simulink model "gsm_sms_sim900_demo"  (Simulink 7.3)
settings: Solver=FixedStepDiscrete  SolverMode=SingleTasking  StartTime=0.0  StopTime=10.0  RelTol=1e-3
PreLoadFcn:
  | waijung.modelPreload; % Required for working with Waijung Blockset. Do not remove.
undefined symbols (not defined in the file): HSEOSC, Link, LQFP176, ST, STM32F417IG
libraries: waijung_atcmd_gsmgprs_lib x2, simulink x1, stm32f4_io_lib x1, stm32f4_adc_lib x1, waijung_string_manipulate x1, stm32f4_device_config_lib x1
CloseFcn:
  | waijung.modelClose; % Required for working with Waijung Blockset. Do not remove.
settings Model: Creator=Krisada  LastModifiedBy=Krisada
settings OptimizationCC: OptimizeModelRefInitCode=on  LifeSpan=1
settings HardwareCC: ProdEndianess=LittleEndian  ProdHWDeviceType=ARM Compatible->Cortex - M4  TargetEndianess=LittleEndian  TargetHWDeviceType=ARM Compatible->Cortex - M4
settings RTWCC: SystemTargetFile=stm32f4.tlc  GenerateMakefile=off  TemplateMakefile=ert_default_tmf  Description=STM32F4 Target  ProcessScript=stm32f4_make_rtw_hook
settings CodeAppCC: IgnoreCustomStorageClasses=off
settings STFCustomTargetCC: ModelReferenceCompliant=off  CombineOutputUpdateFcns=on  ERTCustomFileBanners=on  SupportContinuousTime=off  SupportNonInlinedSFcns=off  SystemTargetFile=stm32f4.tlc
settings ERTTargetCC: MultiwordLength=2048  ModelReferenceCompliant=off  ParMdlRefBuildCompliant=off  CompOptLevelCompliant=off  ERTFirstTimeCompliant=off  ModelStepFunctionPrototypeControlCompliant=off  CPPClassGenCompliant=off  ExtModeMexFile=noextcomm  InlinedParameterPlacement=NonHierarchical  ERTSrcFileBannerTemplate=stm32f4_code_template.cgt  ERTHdrFileBannerTemplate=stm32f4_code_template.cgt  ERTDataSrcFileTemplate=stm32f4_code_template.cgt  ERTDataHdrFileTemplate=stm32f4_code_template.cgt  ERTCustomFileTemplate=stm32f4_file_process.tlc

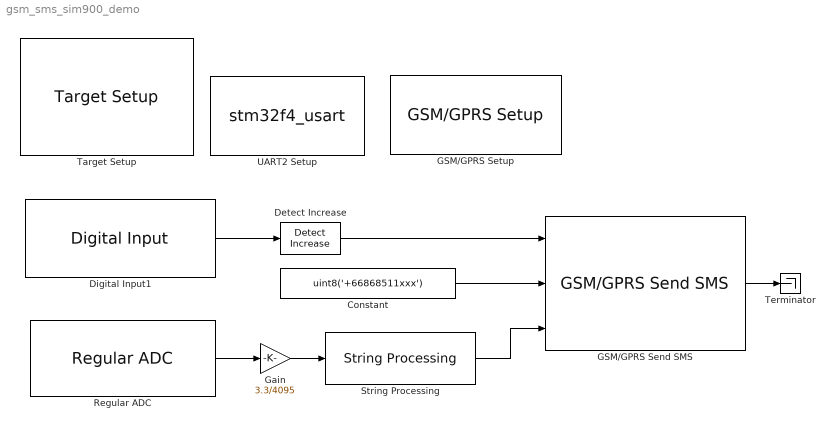
== system gsm_sms_sim900_demo ==
  Constant : Constant  Value=uint8('+66868511xxx')  OutDataType=fixdt(1, 16)  OutScaling=2^0
  Detect Increase : simulink/Logic and Bit Operations/Detect Increase  SystemSampleTime=-1  vinit=0.0
  Digital Input1 : stm32f4_io_lib/Digital Input  port=B  speed=100  porttype=None  porttypestr=NOPULL  use_pin0=off  use_pin1=off  use_pin2=on  use_pin3=off  use_pin4=off  use_pin5=off  use_pin6=off  use_pin7=off  use_pin8=off  use_pin9=off  use_pin10=off  use_pin11=off  use_pin12=off  use_pin13=off  use_pin14=off  use_pin15=off  pinstr=GPIO_Pin_2  usedpinarray="[0  0  1  0  0  0  0  0  0  0  0  0  0  0  0  0]"  bitbandingstr="#define DigitalInput1_B2 Peripheral_BB(GPIOB->IDR, 2)  /* Output pin */"  sampletime=0.01  sampletimestr=0.01  blockid=DigitalInput1  enablecustomportlabel=off  glabalinit=off  cinputportlabel=In1, In2  coutputportlabel=Out1, Out2
  GSM/GPRS Send SMS : waijung_atcmd_gsmgprs_lib/GSM//GPRS Send SMS  conf=SendSMS  portpinstr=0  sampletime=inf  blockid=GSMGPRSSendSMS  inputporttype=[3 3 3]  inputportwidth=[1 -1 -1]  inputportlabel={'Trig','Number','Message'}  outputporttype=[3]  outputportwidth=[1]  outputportlabel={'Status'}  compat=0  optionstring="[\"1\",\"2\",\"GPRS\",\"Internet\",\"D\",\"1\",\"D\",\"0\",\"0\",\"\"]"  stringparam1=''  stringparam2=''
  GSM/GPRS Setup : waijung_atcmd_gsmgprs_lib/GSM//GPRS Setup  conf=Setup  uartmodule=2  connectiontype=GPRS  apn='Internet'  user=''  password=''  pwrkey_port=D  pwrkey_pin=1  reset_port=D  reset_pin=0  portpinstr=0  sampletime=inf  blockid=GSMGPRSSetup  inputporttype=[]  inputportwidth=[]  inputportlabel={}  outputporttype=[]  outputportwidth=[]  outputportlabel={}  compat=0  optionstring="[\"1\",\"2\",\"GPRS\",\"Internet\",\"D\",\"1\",\"D\",\"0\",\"0\",\"\"]"  stringparam1=''  stringparam2=''  stringparam3=''  stringparam4=''
  Gain : Gain  Gain=3.3/4095  ParameterDataType=fixdt(1, 16)  ParameterScaling=2^0  OutDataType=fixdt(1, 16)  OutScaling=2^0
  Regular ADC : stm32f4_adc_lib/Regular ADC  adcmodule=1  outputdatatype=Single  prescaler=2  prescalerstr=ADC_Prescaler_Div2  chsamplingtime=Auto  chsamplingtimestr=ADC_SampleTime_480Cycles  read_an0=off  read_an1=off  read_an2=off  read_an3=off  read_an4=off  read_an5=on  read_an6=off  read_an7=off  read_an8=off  read_an9=off  read_an10=off  read_an11=off  read_an12=off  read_an13=off  read_an14=off  read_an15=off  read_an16=off  read_an17=off  read_an18=off  pinstr=GPIO_Pin_5  usedpinarray="[0  0  0  0  0  1  0  0  0  0  0  0  0  0  0  0  0  0  0]"  usedportidarray=[0]  usedpinidarray=[5]  usedpinidcount=1  sampletime=0.01  blockid=RegularADC  enablecustomportlabel=off  cinputportlabel=0  coutputportlabel=Out1, Out2
  String Processing : waijung_string_manipulate/String Processing  conf=processing  stringfunction=sprintf  stringformat='ADC=%1.2f'  begindelimiter=''  enddelimiter=''  buffersize=64  enablestatus=off  portpinstr=0  sampletime=inf  blockid=StringProcessing  inputporttype=[-1]  inputportwidth=[1]  inputportlabel={'%f'}  outputporttype=[3]  outputportwidth=[64]  outputportlabel={'Output'}  compat=0  optionstring=[]  datatypestring="[\"float\"]"
  Target Setup : stm32f4_device_config_lib/Target Setup  Priority=100  compiler=GNU ARM  previous_compiler=GNU ARM  mcu=STM32F417IG (LQFP176)  mcustr=STM32F417IG  clockconfig=HSEOSC-8MHz  system_stm32f4xx_c_path=F:\trunk\targets\stm32f4_target\stm32f4\utils\system_stm32f4xx_default\STM32F40_41xxx\hseosc8mhz  showmemoryconfiguration=off  stacksize=0x2000  heapsize=0x2000  enableautocompiledownload=on  fullchiperase=off  programmerinterface=ST-Link  editctrlstr=on  compilercontrolstr=$(patsubst %, -I%, .) -mcpu=cortex-m4 -mthumb -mthumb-interwork -mfloat-abi=hard -mfpu=fpv4-sp-d16 -ffast-math -Wall -Wextra -Ofast  assemblercontrolstr=$(patsubst %, -I%, .) -mcpu=cortex-m4 -mthumb -mthumb-interwork -mfloat-abi=hard -mfpu=fpv4-sp-d16 -ffast-math -Wall -Wextra -Ofast -Wa,-amhls=$(<:.s=.lst) -D__STACK_SIZE=$(STACK_SIZE) -D__HEAP_SIZE=$(HEAP_SIZE)  linkercontrolstr=-T$(LD_SCRIPT) -g -Wl,-Map=$(MAP),--cref,--no-warn-mismatch -mcpu=cortex-m4 -mthumb -mthumb-interwork -mfloat-abi=hard -mfpu=fpv4-sp-d16 -specs=nosys.specs  runafterdownload=on  execprofile=None  profileruart=3  profilerbaud=500000  profilertxpin=D8  profilerinitstr=0.01,168000000,1680000,500000,0  manualsetsampletime=off  sampletime=0.01  blockid=TargetSetup  systickreloadvalue=1680000  hseval=8000000  lastprofileruart=3  hclk=168000000  flashorigin=0x8000000  flashlength=1024k  ramorigin=0x20000000  ramlength=128k  useextram=off
  Terminator : Terminator
  UART2 Setup : S-Function  Priority=1  FunctionName=stm32f4_usart  Parameters=configuration,uartmodule,transfer,baudrate,inputtype,outputtype,confstr,binheaderarray,binterminatorarray,asciiheader,asciiterminator,bindatalength,packetmode,varname,sampletime,sampletimestr,blockid  EnableBusSupport=off  mask(stm32f4_usart){configuration=Setup, uartmodule=2, baudrate=115200, databits=8, parity=No, stopbit=1, remaptxpin=D5, remaprxpin=D6, flowcontrol=None, remapctspin=Not used, remaprtspin=Not used, advanceoptions=on, rxbuffersize=2048, txbuffersize=2048, transfer=Blocking, packetmode=Ascii, binheader='7E 7E', binterminator='03 03', porttype_double=1, porttype_single=0, porttype_int8=1, porttype_uint8=0, porttype_int16=0, porttype_uint16=0, porttype_int32=0, porttype_uint32=0, asciiformat='%d,%f', rx_asciiterminator=CRLF (0x0D 0x0A - "\r\n"), tx_asciiterminator=CR (0x0D - "\r"), storagename=<empty>, varname=, inputtype=[0], outputtype=[0], binheaderarray=[0], binterminatorarray=[0], bindatalength=0, asciiheader='', asciiterminator=[0], sampletime=-1, sampletimestr=0.01, blockid=UART2Setup, confstr=[ "dummy", "1", "D", "5", "1", "D", "6", "0", "*", "*", "0", "*", "*", "1", "4", "6", "1", "4", "5", "2048", "2048", "1", "2", "115200", "8", "No", "1", "None", "USART2"], lastmodule=2}
      mask prompts: uartmodule "UART Module"; baudrate "Baud rate (bps)"; databits "Data bits"; stopbit "Stop bit"; remaptxpin "Tx Pin"; remaprxpin "Rx Pin"; flowcontrol "Hardware flow control"; remapctspin "HW Flow control, CTS Pin"; remaprtspin "HW Flow control, RTS Pin"; advanceoptions "Advance options"; rxbuffersize "Rx buffer size (bytes)"; txbuffersize "Tx buffer size (bytes)"; packetmode "Packet mode"; binheader "Binary header (example: '7E 7E')"; binterminator "Binary terminator (example: '03 03')"; porttype_double "Number of data port, type DOUBLE"; porttype_single "Number of data port, type SINGLE"; porttype_int8 "Number of data port, type INT8"; porttype_uint8 "Number of data port, type UINT8"; porttype_int16 "Number of data port, type INT16"; porttype_uint16 "Number of data port, type UINT16"; porttype_int32 "Number of data port, type INT32"; porttype_uint32 "Number of data port, type UINT32"; asciiformat "Ascii format"; rx_asciiterminator "End of packet"; tx_asciiterminator "End of packet"; storagename "Buffer"; varname "Var name"; inputtype "Input data type"; outputtype "Output data type"; binheaderarray "Binary header"; binterminatorarray "Binary terminator"; bindatalength "Binary data length"; asciiheader "Ascii header (printf format)"; asciiterminator "Ascii terminator"; sampletime "Sample time (sec)"; sampletimestr "Compiled sample time (sec) in string"; confstr "Configuration string"; lastmodule "Last module selected"
      mask help:
      | Default STM32F4DISCOVERY + aMG F4 Connect 2 + aMG USB Converter N2 settings use
      |
      | USART3, Tx D8, Rx D9 and USB Serial Converter A.
      mask init:
      | stm32f4_usart_callback('init');
      mask Help: web(fullfile(waijungdocroot,'stm32f4_usart_setup.htm'), '-browser')
      mask StyleString: popup(Setup|Tx|Rx),popup(1|2|3|4|5|6),edit,popup(8),popup(No|Odd|Even),popup(0.5|1|1.5|2),popup(Not used|A2|D5),popup(Not used|A3|D6),popup(None|RTS|CTS|RTS/CTS),popup(Not used|A0|D3),popup(Not used|A1|D4),checkbox,popup(16|32|64|128|256|512|1024|2048),popup(16|32|64|128|256|512|1024|2048),popup(Blocking|Non-Blocking),popup(Ascii|Binary|String Buffer),edit,edit,edit,edit,edit,edit,edit,edit,edit,edit,edit,popup(CR (0x0D - "\r")|LF (0x0A - "\n")|CRLF (0x0D 0x0A - "\r\n")),popup(CR (0x0D - "\r")|LF (0x0A - "\n")|CRLF (0x0D 0x0A - "\r\n")|None),popup(<empty>),edit,edit,edit,edit,edit,edit,edit,edit,edit,edit,edit,edit,edit
      mask CallbackString: stm32f4_usart_callback('configuration');|stm32f4_usart_callback('uartmodule');|stm32f4_usart_callback('baudrate');||||||stm32f4_usart_callback('flowcontrol');|||stm32f4_usart_callback('advanceoptions');|||stm32f4_usart_callback('transfer');|stm32f4_usart_callback('packetmode');|stm32f4_usart_callback('binheader');|stm32f4_usart_callback('binterminator');|stm32f4_usart_callback('porttype');|stm32f4_usart_callback('porttype');|stm32f4_usart_callback('porttype');|stm32f4_usart_callback('porttype');|stm32f4_usart_callback('porttype');|stm32f4_usart_callback('porttype');|stm32f4_usart_callback('porttype');|stm32f4_usart_callback('porttype');|stm32f4_usart_callback('asciiformat');|stm32f4_usart_callback('rx_asciiterminator');|stm32f4_usart_callback('tx_asciiterminator');|stm32f4_usart_callback('storagename');|stm32f4_usart_callback('varname');||||||||stm32f4_usart_callback('sampletime');|stm32f4_usart_callback('sampletimestr');|stm32f4_usart_callback('blockid');||
      mask Display: text(0.5, 0.5, 'Module: USART2_Setup\nBaud (Bps): 115200\nDMA Buffer: 2048/2048\nTx/Rx Pin: D5/D6','ver','middle','hor','center');
  wires:
  Digital Input1/1 -> Detect Increase/1
  Detect Increase/1 -> GSM/GPRS Send SMS/1
  Constant/1 -> GSM/GPRS Send SMS/2
  String Processing/1 -> GSM/GPRS Send SMS/3
  Regular ADC/1 -> Gain/1
  Gain/1 -> String Processing/1
  GSM/GPRS Send SMS/1 -> Terminator/1
